simulink model "path_following_3d"  (R2023b)
settings: Solver=VariableStepAuto  StartTime=0.0  StopTime=10.0  RelTol=1e-3
values from neighbouring files (symbols this model uses):
  g = 9.8    [para.m]
  m = 2    [para.m]
  n = n/norm(n)    [para.m]
  P = [0;1;-3]    [para.m]
  vd = 3    [para.m]
libraries: shared6dof x1
settings Model: Creator=arthus  LastModifiedBy=kevin
settings SolverCC: AlgebraicLoopSolver=TrustRegion
settings DataIOCC: ReturnWorkspaceOutputs=off
settings DebuggingCC: UnconnectedInputMsg=warning  UnconnectedOutputMsg=warning  UnconnectedLineMsg=warning  ArithmeticOperatorsInVariantConditions=warning
settings ModelReferenceCC: EnableRefExpFcnMdlSchedulingChecks=on
settings SFSimCC: CustomCodeUndefinedFunction=UseInterfaceOnly

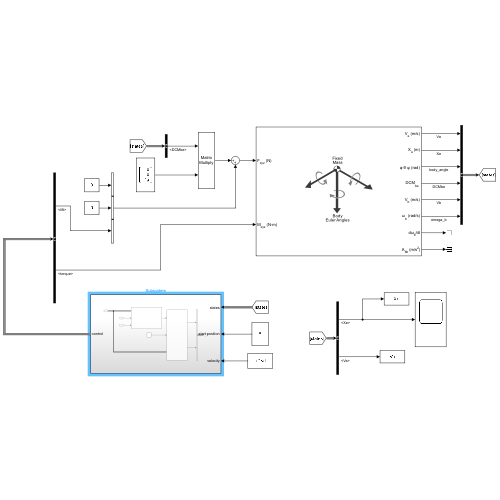
[thumbnail: Simulink's stored preview of the top-level diagram]
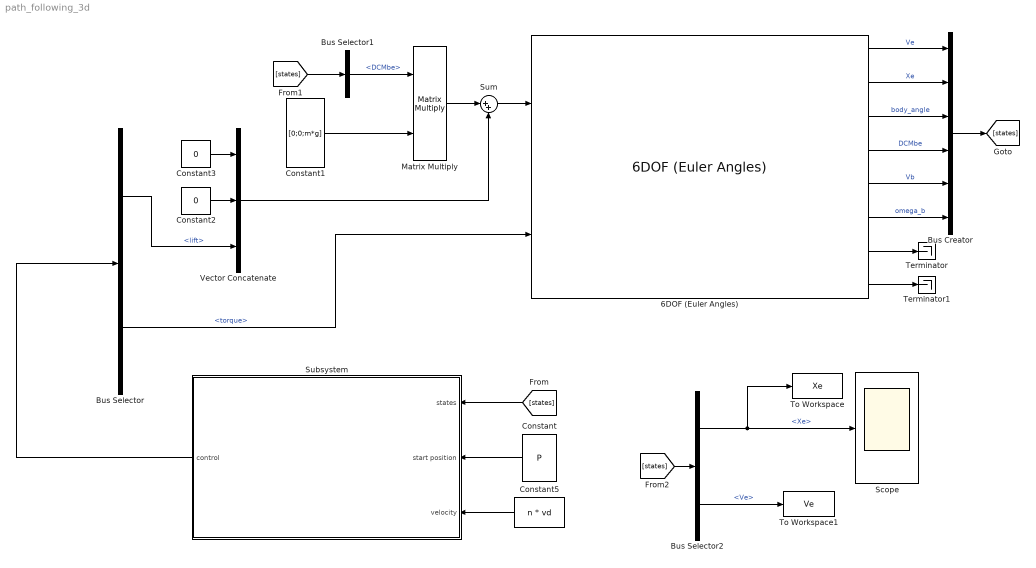
== system path_following_3d ==
  6DOF (Euler Angles) : shared6dof/6DOF (Euler Angles)  units=Metric (MKS)  mtype=Fixed  rep=Euler Angles  xme_0=[0 0 0]  Vm_0=[0 0 0]  eul_0=[0 0 0]  pm_0=[0 0 0]  mass_0=m  mass_e=0.5  mass_f=2.0  inertia=J  inertia_e=eye(3)  inertia_f=2*eye(3)  k_quat=1.0  vre_flag=on  abi_flag=off  aMode=0  xme_statename=''  Vm_statename=''  eul_statename=''  quat_statename=''  pm_statename=''  mass_statename=''
  Bus Creator : BusCreator  Inputs=6
  Bus Selector : BusSelector  OutputSignals=lift,torque
  Bus Selector1 : BusSelector  OutputSignals=DCMbe
  Bus Selector2 : BusSelector  OutputSignals=Xe,Ve
  Constant : Constant  Value=P  VectorParams1D=off
  Constant1 : Constant  Value=[0;0;m*g]  VectorParams1D=off
  Constant2 : Constant  Value=0  VectorParams1D=off
  Constant3 : Constant  Value=0  VectorParams1D=off
  Constant5 : Constant  Value=n * vd  VectorParams1D=off
  Matrix Multiply : Product  Multiplication=Matrix(*)
  Scope : Scope
  Subsystem : Subsystem
  Sum : Sum  Inputs=|++
  Terminator : Terminator
  Terminator1 : Terminator
  To Workspace : ToWorkspace  VariableName=Xe  SaveFormat=Timeseries  SampleTime=-1
  To Workspace1 : ToWorkspace  VariableName=Ve  SaveFormat=Timeseries  SampleTime=-1
  Vector Concatenate : Concatenate  NumInputs=3
  wires:
  6DOF (Euler Angles)/7 -> Terminator/1
  6DOF (Euler Angles)/8 -> Terminator1/1
  6DOF (Euler Angles)/6 -> Bus Creator/6  "omega_b"
  6DOF (Euler Angles)/5 -> Bus Creator/5  "Vb"
  6DOF (Euler Angles)/4 -> Bus Creator/4  "DCMbe"
  6DOF (Euler Angles)/3 -> Bus Creator/3  "body_angle"
  6DOF (Euler Angles)/2 -> Bus Creator/2  "Xe"
  6DOF (Euler Angles)/1 -> Bus Creator/1  "Ve"
  Bus Creator/1 -> [states]
  [states] -> Subsystem/1(states)
  Constant/1 -> Subsystem/2(start position)
  Subsystem/1(control) -> Bus Selector/1
  Bus Selector/2 -> 6DOF (Euler Angles)/2  "<torque>"
  Constant1/1 -> Matrix Multiply/2
  [states] -> Bus Selector1/1
  Bus Selector1/1 -> Matrix Multiply/1  "<DCMbe>"
  Sum/1 -> 6DOF (Euler Angles)/1
  Matrix Multiply/1 -> Sum/1
  Vector Concatenate/1 -> Sum/2
  Constant2/1 -> Vector Concatenate/2
  Constant3/1 -> Vector Concatenate/1
  Bus Selector/1 -> Vector Concatenate/3  "<lift>"
  [states] -> Bus Selector2/1
  Bus Selector2/1 -> To Workspace/1, Scope/1  "<Xe>"
  Constant5/1 -> Subsystem/3(velocity)
  Bus Selector2/2 -> To Workspace1/1  "<Ve>"

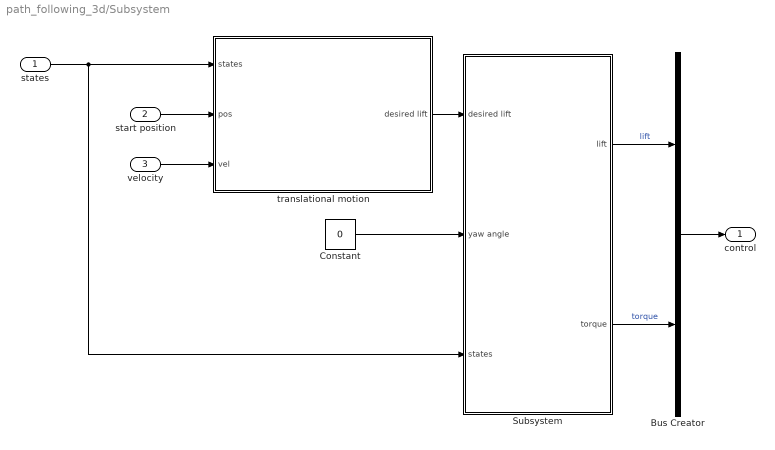
== system path_following_3d/Subsystem ==
  states : Inport
  start position : Inport  Port=2
  velocity : Inport  Port=3
  Bus Creator : BusCreator  Inputs=2
  Constant : Constant  Value=0
  Subsystem : Subsystem
  translational motion : Subsystem
  control : Outport  VectorParamsAs1DForOutWhenUnconnected=off
  wires:
  translational motion/1(desired lift) -> Subsystem/1(desired lift)
  Constant/1 -> Subsystem/2(yaw angle)
  states/1 -> Subsystem/3(states), translational motion/1(states)
  start position/1 -> translational motion/2(pos)
  Subsystem/2(torque) -> Bus Creator/2  "torque"
  Subsystem/1(lift) -> Bus Creator/1  "lift"
  Bus Creator/1 -> control/1
  velocity/1 -> translational motion/3(vel)

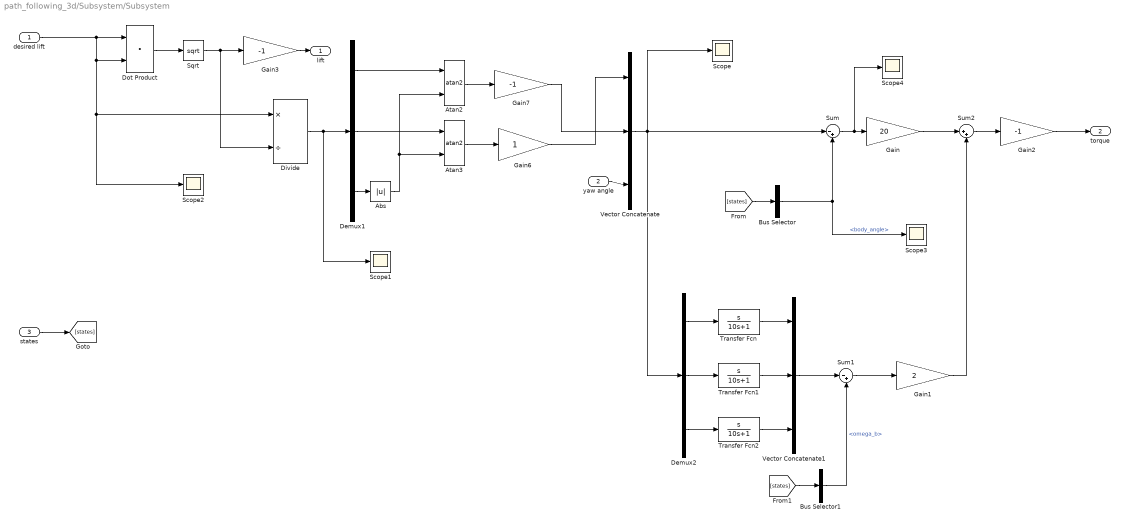
== system path_following_3d/Subsystem/Subsystem ==
  desired lift : Inport
  yaw angle : Inport  Port=2
  states : Inport  Port=3
  Abs : Abs  SaturateOnIntegerOverflow=off
  Atan2 : Trigonometry  Operator=atan2
  Atan3 : Trigonometry  Operator=atan2
  Bus Selector : BusSelector  OutputSignals=body_angle
  Bus Selector1 : BusSelector  OutputSignals=omega_b
  Demux1 : Demux  Outputs=3
  Demux2 : Demux  Outputs=3
  Divide : Product  Inputs=*/
  Dot Product : DotProduct  OutDataTypeStr=Inherit: Inherit via internal rule
  Gain : Gain  Gain=20
  Gain1 : Gain  Gain=2
  Gain2 : Gain  Gain=-1
  Gain3 : Gain  Gain=-1
  Gain6 : Gain
  Gain7 : Gain  Gain=-1
  Scope{,1..4} (5 alike) : Scope
  Sqrt : Sqrt
  Sum : Sum  Inputs=|-+
  Sum1 : Sum  Inputs=|-+
  Sum2 : Sum  Inputs=|++
  Transfer Fcn : TransferFcn  Numerator=[1 0]  Denominator=[10 1]
  Transfer Fcn1 : TransferFcn  Numerator=[1 0]  Denominator=[10 1]
  Transfer Fcn2 : TransferFcn  Numerator=[1 0]  Denominator=[10 1]
  Vector Concatenate : Concatenate  NumInputs=3
  Vector Concatenate1 : Concatenate  NumInputs=3
  lift : Outport  VectorParamsAs1DForOutWhenUnconnected=off
  torque : Outport  Port=2  VectorParamsAs1DForOutWhenUnconnected=off
  wires:
  states/1 -> [states]
  [states] -> Bus Selector/1
  Bus Selector/1 -> Scope3/1, Sum/2  "<body_angle>"
  Sqrt/1 -> Divide/2, Gain3/1
  Dot Product/1 -> Sqrt/1
  desired lift/1 -> Scope2/1, Divide/1, Dot Product/2, Dot Product/1
  Divide/1 -> Scope1/1, Demux1/1
  yaw angle/1 -> Vector Concatenate/3
  Sum2/1 -> Gain2/1
  Gain2/1 -> torque/1
  Bus Selector1/1 -> Sum1/2  "<omega_b>"
  Sum1/1 -> Gain1/1
  Gain1/1 -> Sum2/2
  Gain/1 -> Sum2/1
  Sum/1 -> Scope4/1, Gain/1
  Vector Concatenate/1 -> Scope/1, Demux2/1, Sum/1
  [states] -> Bus Selector1/1
  Gain3/1 -> lift/1
  Vector Concatenate1/1 -> Sum1/1
  Transfer Fcn/1 -> Vector Concatenate1/1
  Transfer Fcn1/1 -> Vector Concatenate1/2
  Transfer Fcn2/1 -> Vector Concatenate1/3
  Demux2/1 -> Transfer Fcn/1
  Demux2/2 -> Transfer Fcn1/1
  Demux2/3 -> Transfer Fcn2/1
  Demux1/1 -> Atan2/1
  Demux1/3 -> Abs/1
  Demux1/2 -> Atan3/1
  Atan3/1 -> Gain6/1
  Atan2/1 -> Gain7/1
  Gain6/1 -> Vector Concatenate/1
  Gain7/1 -> Vector Concatenate/2
  Abs/1 -> Atan3/2, Atan2/2

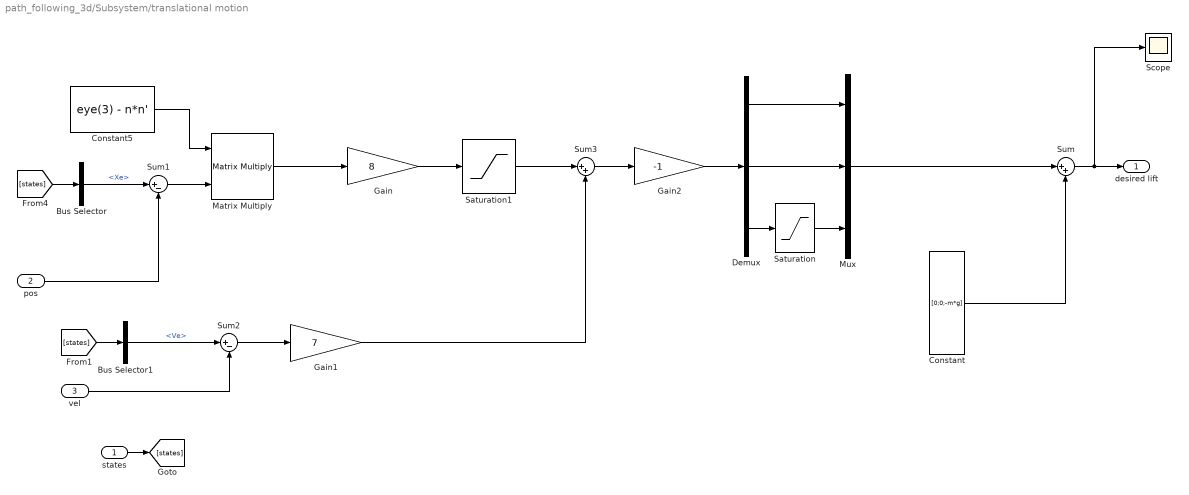
== system path_following_3d/Subsystem/translational motion ==
  states : Inport
  pos : Inport  Port=2
  vel : Inport  Port=3
  Bus Selector : BusSelector  OutputSignals=Xe
  Bus Selector1 : BusSelector  OutputSignals=Ve
  Constant : Constant  Value=[0;0;-m*g]  VectorParams1D=off
  Constant5 : Constant  Value=eye(3) - n*n'  VectorParams1D=off
  Demux : Demux  Outputs=3
  Gain : Gain  Gain=8
  Gain1 : Gain  Gain=7
  Gain2 : Gain  Gain=-1
  Matrix Multiply : Product  Multiplication=Matrix(*)
  Mux : Mux  Inputs=3
  Saturation : Saturate  UpperLimit=0.9 * m * g  LowerLimit=-inf
  Saturation1 : Saturate  UpperLimit=5  LowerLimit=-5
  Scope : Scope
  Sum : Sum  Inputs=|++
  Sum1 : Sum  Inputs=|+-
  Sum2 : Sum  Inputs=|+-
  Sum3 : Sum  Inputs=|++
  desired lift : Outport  VectorParamsAs1DForOutWhenUnconnected=off
  wires:
  Sum/1 -> Scope/1, desired lift/1
  Constant/1 -> Sum/2
  Gain2/1 -> Demux/1
  Gain/1 -> Saturation1/1
  Demux/1 -> Mux/1
  Sum3/1 -> Gain2/1
  Gain1/1 -> Sum3/2
  pos/1 -> Sum1/2
  states/1 -> [states]
  [states] -> Bus Selector/1
  Bus Selector/1 -> Sum1/1  "<Xe>"
  [states] -> Bus Selector1/1
  Demux/2 -> Mux/2
  Mux/1 -> Sum/1
  Demux/3 -> Saturation/1
  Saturation/1 -> Mux/3
  Bus Selector1/1 -> Sum2/1  "<Ve>"
  vel/1 -> Sum2/2
  Sum2/1 -> Gain1/1
  Saturation1/1 -> Sum3/1
  Constant5/1 -> Matrix Multiply/1
  Matrix Multiply/1 -> Gain/1
  Sum1/1 -> Matrix Multiply/2
